simulink model "FSK_EXP3"  (R2020a)
settings: Solver=VariableStepAuto  StartTime=0.0  StopTime=20  RelTol=1e-3
libraries: commrandsrc3 x1, dsparch4 x1
settings Model: Creator=User  LastModifiedBy=Raksha

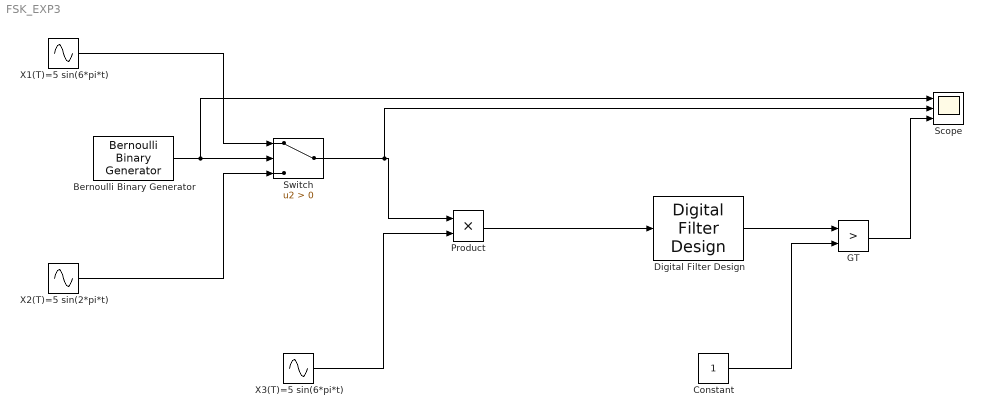
== system FSK_EXP3 ==
  Bernoulli Binary Generator : commrandsrc3/Bernoulli Binary Generator  ProbabilityOfZero=0.5  SeedSource=Auto  Seed=0  SampleTime=1  SamplesPerFrame=1  OutputDataType=double  SimulateUsing=Interpreted execution
  Constant : Constant
  Digital Filter Design : dsparch4/Digital Filter Design  mwdsp_browser_bugfix_var=off
  GT : RelationalOperator  Operator=>  OutDataTypeStr=boolean  RndMeth=Simplest
  Product : Product
  Scope : Scope  NumInputPorts=3
  Switch : Switch  Criteria=u2 > Threshold
  X1(T)=5 sin(6*pi*t) : Sin  Amplitude=5  Frequency=6*pi  SampleTime=0.01
  X2(T)=5 sin(2*pi*t) : Sin  Amplitude=5  Frequency=2*pi  SampleTime=0.01
  X3(T)=5 sin(6*pi*t) : Sin  Amplitude=5  Frequency=6*pi  SampleTime=0.1
  wires:
  Bernoulli Binary Generator/1 -> Scope/1, Switch/2
  X1(T)=5 sin(6*pi*t)/1 -> Switch/1
  X2(T)=5 sin(2*pi*t)/1 -> Switch/3
  X3(T)=5 sin(6*pi*t)/1 -> Product/2
  Switch/1 -> Scope/2, Product/1
  Product/1 -> Digital Filter Design/1
  Constant/1 -> GT/2
  Digital Filter Design/1 -> GT/1
  GT/1 -> Scope/3
